simulink model "prbs_model"  (R2022a)
settings: Solver=ode4  StartTime=0.0  StopTime=4.096  FixedStep=1e-3  RelTol=1e-3
libraries: dspsrcs4 x1, discretizing x1
settings Model: Creator=randolf  LastModifiedBy=randolf
settings OptimizationCC: DefaultParameterBehavior=Inlined  UseDivisionForNetSlopeComputation=on  GainParamInheritBuiltInType=on  UseFloatMulNetSlope=on  InlineInvariantSignals=on  PassReuseOutputArgsAs=Individual arguments  ZeroExternalMemoryAtStartup=off  ZeroInternalMemoryAtStartup=off  NoFixptDivByZeroProtection=on  EfficientFloat2IntCast=on  LifeSpan=1  OptimizeBlockOrder=speed  DifferentSizesBufferReuse=on  EfficientTunableParamExpr=on
settings DebuggingCC: ParameterTunabilityLossMsg=error
settings HardwareCC: ProdBitPerPointer=32  ProdBitPerSizeT=32  ProdBitPerPtrDiffT=32  ProdLargestAtomicInteger=Long  ProdLargestAtomicFloat=Double  ProdWordSize=32  ProdLongLongMode=on  ProdHWDeviceType=ARM Compatible->ARM Cortex-M
settings SFSimCC: MATLABDynamicMemAlloc=off
settings RTWCC: SystemTargetFile=ert.tlc  TemplateMakefile=ert_default_tmf
settings CodeAppCC: ForceParamTrailComments=on  IgnoreCustomStorageClasses=off  OperatorAnnotations=on  SimulinkDataObjDesc=on  SFDataObjDesc=on  CustomSymbolStrGlobalVar=rt$N$M  CustomSymbolStrType=$N$M  CustomSymbolStrFcn=$N$M$F  CustomSymbolStrMacro=$N$M  InsertBlockDesc=on
settings ERTTargetCC: TargetLangStandard=C99 (ISO)  GenerateSampleERTMain=on  IncludeMdlTerminateFcn=off  CombineSignalStateStructs=on  SupportComplex=off  SupportNonInlinedSFcns=on  InlinedParameterPlacement=NonHierarchical  ERTCustomFileTemplate=example_file_process.tlc  ERTFilePackagingFormat=CompactWithDataFile

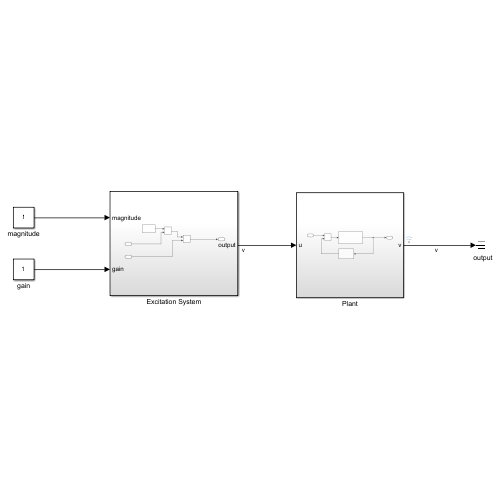
[thumbnail: Simulink's stored preview of the top-level diagram]
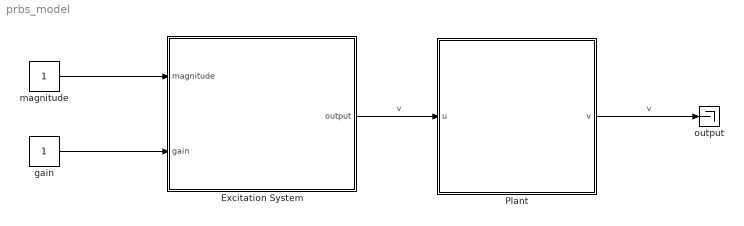
== system prbs_model ==
  Excitation System : Subsystem
  Plant : Subsystem
  gain : Constant
  magnitude : Constant
  output : Terminator
  wires:
  magnitude/1 -> Excitation System/1(magnitude)
  gain/1 -> Excitation System/2(gain)
  Plant/1(v) -> output/1  "v"
  Excitation System/1(output) -> Plant/1(u)  "v"

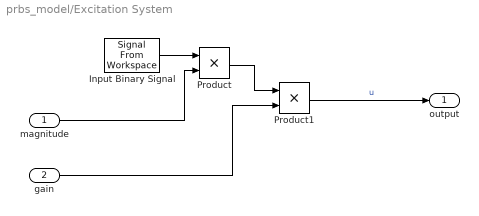
== system prbs_model/Excitation System ==
  magnitude : Inport
  gain : Inport  Port=2
  Input Binary Signal : dspsrcs4/Signal From Workspace  X=binary_signal  Ts=0.001  nsamps=1  OutputAfterFinalValue=Setting to zero  ignoreOrWarnInputAndFrameLengths=off  OutputFrames=off
  Product : Product
  Product1 : Product
  output : Outport
  wires:
  Input Binary Signal/1 -> Product/1
  Product/1 -> Product1/1
  gain/1 -> Product1/2
  magnitude/1 -> Product/2
  Product1/1 -> output/1  "u"

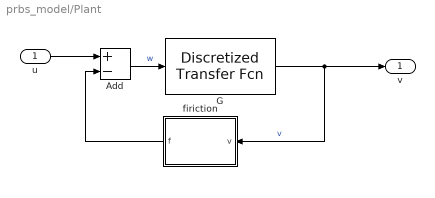
== system prbs_model/Plant ==
  u : Inport
  Add : Sum  Inputs=+-
  G : discretizing/Discretized Transfer Fcn  Numerator=[10]  Denominator=[1 10]  AbsTol=auto  SampleTime=1e-3  method=zoh  Wc=1
      settings: SourceProductBaseCode=SL
  firiction : MATLAB Function  TreatAsAtomicUnit=on
  v : Outport
  wires:
  u/1 -> Add/1
  G/1 -> v/1, firiction/1(v)  "v"
  Add/1 -> G/1  "w"
  firiction/1(f) -> Add/2

== matlab function prbs_model/Plant/firiction ==
  data: v input; f output
function f = fcn(v)
    if (v>0)
        f = 0.5;
    else
        f = -0.4;
    end
end
